simulink model "linio_nochmal_nur_CC2"  (R2013a)
settings: Solver=ode45  StartTime=0.0  StopTime=1e-3  MaxStep=10e-7  RelTol=1e-3
InitFcn:
  | param=evalin('base','param;');
  | 
  | JR=str2num(param.JR);
  | KMT=str2num(param.KMT);
  | Rc=str2num(param.Rc);
  | Lc=str2num(param.Lc);
  | KFR=str2num(param.KFR);
  | KTB=str2num(param.KTB);
  | KBM=str2num(param.KBM);
  | Rsh=str2num(param.Rsh);
StartFcn:
  | %sprintf('Info (%s):\nKTB = %.1e\nKBM = %.1e\n', gcs, KTB, KBM)
libraries: simulink x1
settings Model: Creator=mainster  LastModifiedBy=mainster

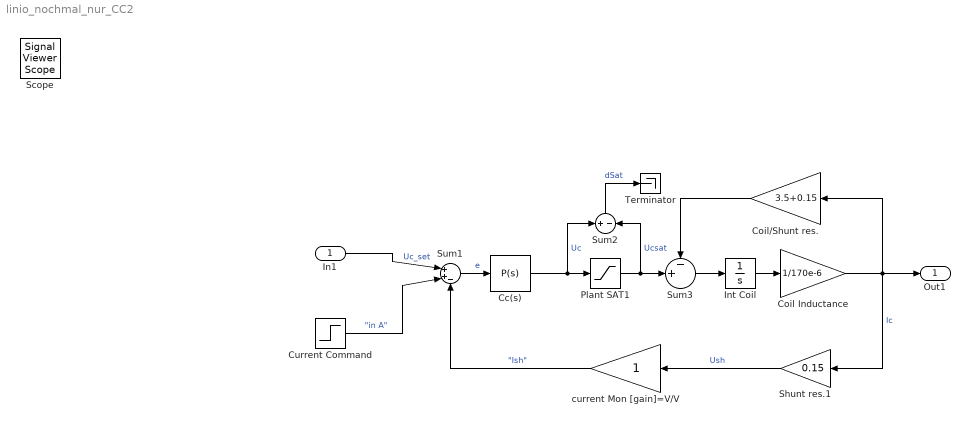
== system linio_nochmal_nur_CC2 ==
  In1 : Inport
  Cc(s) : simulink/Continuous/PID Controller  Controller=P  TimeDomain=Continuous-time  SampleTime=-1  IntegratorMethod=Forward Euler  FilterMethod=Forward Euler  Form=Ideal  P=5  I=14078.2261040339  D=0  N=100  InitialConditionSource=internal  InitialConditionForIntegrator=0  InitialConditionForFilter=0  ExternalReset=none  LimitOutput=off  UpperSaturationLimit=inf  LowerSaturationLimit=-inf  LinearizeAsGain=on  AntiWindupMode=none  Kb=1  TrackingMode=off  Kt=1  PParamMin=[]  PParamMax=[]  IParamMin=[]  IParamMax=[]  DParamMin=[]  DParamMax=[]  NParamMin=[]  NParamMax=[]  KbParamMin=[]  KbParamMax=[]  KtParamMin=[]  KtParamMax=[]  POutMin=[]  POutMax=[]  IOutMin=[]  IOutMax=[]  DOutMin=[]  DOutMax=[]  NOutMin=[]  NOutMax=[]  KbOutMin=[]  KbOutMax=[]  KtOutMin=[]  KtOutMax=[]  IntegratorOutMin=[]  IntegratorOutMax=[]  FilterOutMin=[]  FilterOutMax=[]  SumOutMin=[]  SumOutMax=[]  SumI1OutMin=[]  SumI1OutMax=[]  SumI2OutMin=[]  SumI2OutMax=[]  SumI3OutMin=[]  SumI3OutMax=[]  SumDOutMin=[]  SumDOutMax=[]  SaturationOutMin=[]  SaturationOutMax=[]  IntegratorContinuousStateAttributes=''  IntegratorStateMustResolveToSignalObject=off  IntegratorRTWStateStorageClass=Auto  FilterContinuousStateAttributes=''  FilterStateMustResolveToSignalObject=off  FilterRTWStateStorageClass=Auto
  Coil Inductance : Gain  Gain=1/170e-6
  Coil/Shunt res. : Gain  Gain=3.5+0.15
  Current Command : Step  Time=0.3e-3  SampleTime=0
  Int Coil : Integrator
  Plant SAT1 : Saturate  UpperLimit=25  LowerLimit=-25
      settings: AttributesFormatString=U_lim=+-%<UpperLimit>V
  Shunt res.1 : Gain  Gain=0.15
  Sum1 : Sum  Inputs=|++-
  Sum2 : Sum  Inputs=+-
  Sum3 : Sum  Inputs=-+|
  Terminator : Terminator
  current Mon [gain]=V/V : Gain
  Out1 : Outport
  Scope : SignalViewerScope  IOType=viewer  NumInputPorts=5  LegendLocations=|  RefreshTime=0.035000
      | 0.85952     0.92887     0.14009    0.024213
      | 0.78522     0.72231      0.1308     0.04313
      | 0.85952     0.55357     0.14009     0.04313
      | 0.85023     0.36592     0.11223    0.024213
      |  0.8363     0.17827     0.12152    0.024213
      settings: ShowLegends=on  TimeRange=0.001  YMin=0~0~0~0~-1  YMax=5~25~5~0.08~1
  wires:
  In1/1 -> Sum1/1  "Uc_set"
  Sum1/1 -> Cc(s)/1  "e"
  Coil Inductance/1 -> Shunt res.1/1, Out1/1, Coil/Shunt res./1  "Ic"
  Coil/Shunt res./1 -> Sum3/1
  Sum3/1 -> Int Coil/1
  Int Coil/1 -> Coil Inductance/1
  Cc(s)/1 -> Sum2/1, Plant SAT1/1  "Uc"
  Shunt res.1/1 -> current Mon [gain]=V/V/1  "Ush"
  current Mon [gain]=V/V/1 -> Sum1/3  "\"Ish\""
  Plant SAT1/1 -> Sum2/2, Sum3/2  "Ucsat"
  Current Command/1 -> Sum1/2  "\"in A\""
  Sum2/1 -> Terminator/1  "dSat"
